simulink model "tut6_blackbox"  (Simulink 7.4)
settings: Solver=ode45  StartTime=0.0  StopTime=10.0  RelTol=1e-3
undefined symbols (not defined in the file or in its folder): gcbh, xlBlockLoadCallback
libraries: xbsIndex_r4 x4, xps_library x4, casper_library_misc x2
settings Model: Creator=jack  LastModifiedBy=jack

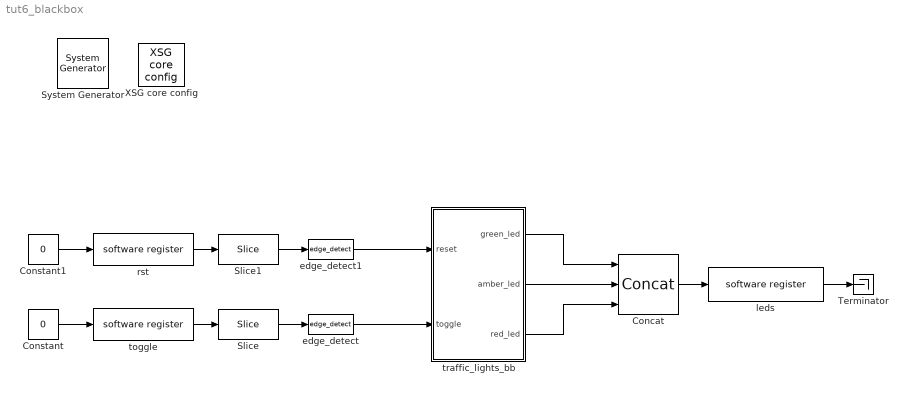
== system tut6_blackbox ==
  " System Generator" : xbsIndex_r4/ System Generator  Tag=genX  SystemSampleTime=-1  xilinxfamily=virtex5  part=xc5vsx95t  speed=-1  package=ff1136  synthesis_tool=XST  clock_wrapper=Clock Enables  directory=./tut6_blackbox/sysgen  testbench=off  simulink_period=1  sysclk_period=10  dcm_input_clock_period=100  incr_netlist=off  trim_vbits=Everywhere in SubSystem  dbl_ovrd=According to Block Masks  core_generation=According to Block Masks  run_coregen=off  deprecated_control=off  eval_field=0  block_type=sysgen
      settings: block_version=11.4
  Concat : xbsIndex_r4/Concat  num_inputs=3  dbl_ovrd=off  block_type=concat
  Constant : Constant  Value=0  OutDataType=fixdt(1, 16)  OutScaling=2^0
  Constant1 : Constant  Value=0  OutDataType=fixdt(1, 16)  OutScaling=2^0
  Slice : xbsIndex_r4/Slice  nbits=1  boolean_output=on  mode=Lower Bit Location + Width  bit1=0  base1=MSB of Input  bit0=0  base0=LSB of Input  dbl_ovrd=off  block_type=slice
  Slice1 : xbsIndex_r4/Slice  nbits=1  boolean_output=on  mode=Lower Bit Location + Width  bit1=0  base1=MSB of Input  bit0=0  base0=LSB of Input  dbl_ovrd=off  block_type=slice
  Terminator : Terminator
  XSG core config : xps_library/XSG core config  Tag=xps:xsg  SystemSampleTime=-1  hw_sys=ROACH:sx95t  ibob_linux=off  clk_src=sys_clk  iBOB_clk_src=sys_clk  BEE2_ctrl_clk_src=sys_clk  BEE2_usr_clk_src=sys_clk  ROACH_clk_src=sys_clk  ROACH2_clk_src=adc0_clk  CORR_clk_src=sys_clk  gpio_clk_io_group=iBOB:sma  gpio_clk_bit_index=0  clk_rate=100  sample_period=1  synthesis_tool=XST  mpc_type=powerpc440_ext
  edge_detect : casper_library_misc/edge_detect  SystemSampleTime=-1  edge=Rising  polarity=Active High  x_in=[0 0.08 0.08 0.16 0.16 0.24 0.24 0.32 0.32 0.4]  y_in="[-1 -1  1  1  1  1  1  1  1  1]"  x_out=[0.6 0.68 0.68 0.76 0.76 0.84 0.84 0.92 0.92 1]  y_out="[-1 -1  1  1 -1 -1 -1 -1 -1 -1]"
  edge_detect1 : casper_library_misc/edge_detect  SystemSampleTime=-1  edge=Rising  polarity=Active High  x_in=[0 0.08 0.08 0.16 0.16 0.24 0.24 0.32 0.32 0.4]  y_in="[-1 -1  1  1  1  1  1  1  1  1]"  x_out=[0.6 0.68 0.68 0.76 0.76 0.84 0.84 0.92 0.92 1]  y_out="[-1 -1  1  1 -1 -1 -1 -1 -1 -1]"
  leds : xps_library/software register  Tag=xps:sw_reg  SystemSampleTime=-1  io_dir=To Processor  arith_type=Unsigned  bitwidth=32  bin_pt=0  sample_period=1  gw_name=tut6_blackbox_leds_user_data_in
  rst : xps_library/software register  Tag=xps:sw_reg  SystemSampleTime=-1  io_dir=From Processor  arith_type=Unsigned  bitwidth=32  bin_pt=0  sample_period=1  gw_name=tut6_blackbox_rst_user_data_out
  toggle : xps_library/software register  Tag=xps:sw_reg  SystemSampleTime=-1  io_dir=From Processor  arith_type=Unsigned  bitwidth=32  bin_pt=0  sample_period=1  gw_name=tut6_blackbox_toggle_user_data_out
  traffic_lights_bb : Subsystem  mask{amber_time=200000000}
      mask prompts: amber_time "Number of amber light clock cycles?"
  wires:
  toggle/1 -> Slice/1
  Slice/1 -> edge_detect/1
  edge_detect/1 -> traffic_lights_bb/2(toggle)
  rst/1 -> Slice1/1
  Slice1/1 -> edge_detect1/1
  edge_detect1/1 -> traffic_lights_bb/1(reset)
  Concat/1 -> leds/1
  traffic_lights_bb/1(green_led) -> Concat/1
  traffic_lights_bb/2(amber_led) -> Concat/2
  traffic_lights_bb/3(red_led) -> Concat/3
  leds/1 -> Terminator/1
  Constant/1 -> toggle/1
  Constant1/1 -> rst/1

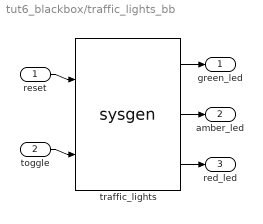
== system tut6_blackbox/traffic_lights_bb ==
  reset : Inport
  toggle : Inport  Port=2
  traffic_lights : S-Function  AncestorBlock=xbsIndex_r4/Black Box  LoadFcn=xlBlockLoadCallback(gcbh);  FunctionName=sysgen  Parameters=ptable_  EnableBusSupport=off  mask(Xilinx Black Box Block){infoedit=Incorporates black box HDL and simulation model into a System Generator design.<br><br>You must supply a Black Box with certain information about the HDL component you would like to bring into System Generator. This information is provided through a Matlab function.<br><br>When "Simulation mode" is set to "Inactive", you will typically want to provide a separate simulation model by using a Simulation Multiplexer.<br>When "Simulation mode" is set to "External co-simulator", you must include a ModelSim block in the design., init_code=traffic_lights_config, sim_method_sgadvanced=, sim_method=ISE Simulator, engine_block=, verbose=off, xl_use_area_sgadvanced=, xl_use_area=off, xl_area=[0,0,0,0,0,0,0], has_advanced_control=0, sggui_pos=1300,29,399,477, block_type=blackbox2, block_version=11.4, sg_icon_stat=105,152,2,3,white,blue,0,ffa1fd99,right,, sg_mask_display=|, sg_list_contents={'table'=>{'sim_method'=>'popup(Inactive|ISE Simulator|External co-simulator)','userSelections'=>{'sim_method'=>'ISE Simulator'}}}, sg_blockgui_xml=, amber_time=amber_time}
      mask sg_mask_display=|
      | fprintf('','COMMENT: begin icon graphics');
      | patch([0 1 1 0 ],[0 0 1 1 ],[0.77 0.82 0.91]);
      | patch([0.228571 0.0666667 0.304762 0.0666667 0.228571 0.495238 0.571429 0.647619 0.933333 0.714286 0.504762 0.352381 0.590476 0.352381 0.504762 0.714286 0.933333 0.647619 0.571429 0.495238 0.228571 ],[0.230263 0.342105 0.506579 0.671053 0.782895 0.782895 0.730263 0.782895 0.782895 0.631579 0.776316 0.671053 0.506579 0.342105 0.236842 0.381579 0.230263 0.230263 0.282895 0.230263 0.230263 ],[0.98 0.96 0.92]);
      | plot([0 1 1 0 0 ],[0 0 1 1 0 ]);
      | fprintf('','COMMENT: end icon graphics');
      | fprintf('','COMMENT: begin icon text');
      | color('black');port_label('input',1,'reset');
      | color('black');port_label('input',2,'toggle');
      | color('black');port_label('output',1,'green_led');
      | color('black');port_label('output',2,'amber_led');
      | color('black');port_label('output',3,'red_led');
      | fprintf('','COMMENT: end icon text');
      mask prompts: infoedit ""; init_code "Block configuration m-function"; sim_method_sgadvanced ""; sim_method "Simulation mode"; engine_block "HDL co-simulator to use  (specify helper block by name)"; xl_use_area_sgadvanced ""; xl_use_area "Define FPGA area for resource estimation"; xl_area "FPGA area [slices, FFs, BRAMs, LUTs, IOBs, emb. mults, TBUFs]"; has_advanced_control ""; sggui_pos ""; block_type ""; block_version ""; sg_icon_stat ""; sg_mask_display ""; sg_list_contents ""; sg_blockgui_xml ""; amber_time "Amber clock light cycles?"
      mask help:
      | Incorporates black box HDL and simulation model into a System Generator design.
      |
      | You must supply a Black Box with certain information about the HDL component you would like to bring into System Generator. This information is provided through a Matlab function.
      |
      | When "Simulation mode" is set to "Inactive", you will typically want to provide a separate simulation model by using a Simulation Multiplexer.
      | When "Simulation mode" is set to "External co-simulator", you must include a ModelSim block in the design.
      mask init:
      | try
      |   tmp_gcb = gcb;
      |   tmp_gcbh = gcbh;
      |   if (strcmp('SysGenIndex',get_param(bdroot(tmp_gcbh),'tag')) && ~isempty(regexp(bdroot(tmp_gcb), '^xbs', 'once')))
      |     return;
      |   end;
      |   xlMungeMaskParams;
      |   block_config = 'sysgen_blockset:black_box_config';
      | 
      |   block_type='blackbox2';
      | 
      |   serialized_declarations = '{''engineWorkDir''=>''String'',''engine_block''=>''String'',''engine_handle''=>''Double'',''init_code''=>''String'',''mdlPath''=>''String'',''sim_method''=>''Int'',''srcPath''=>''String'',''validEngineBlock''=>''Int'',''verbose''=>''Bool'',''block_type''=>''String''}';
      |   xlblackbox2_init();
      |   ptable_ = xlblockprep(get_param(tmp_gcb, 'MaskWSVariables'));
      | catch
      |   global dbgsysgen;
      |   if(~isempty(dbgsysgen) && dbgsysgen)
      |     e = regexprep(lasterr, '\n', '\nError: ');
      |     disp(['Error: While running MaskInit code on block ' tmp_gcb ': ' e]);
      |     error(e);
      |   end
      | end
      settings: CopyFcn=xlBlockMoveCallback(gcbh);;xlbbCopyCallback;  DeleteFcn=xlDestroyGui(gcbh);  ModelCloseFcn=xlDestroyGui(gcbh);  PreSaveFcn=xlBlockPreSaveCallback(gcbh);  PostSaveFcn=xlBlockPostSaveCallback(gcbh);  DestroyFcn=xlDestroyGui(gcbh);  OpenFcn=xlOpenGui(gcbh, 'blackbox2_gui.xml', @blackbox2enablement, -1)  CloseFcn=xlDestroyGui(gcbh);  MoveFcn=xlBlockMoveCallback(gcbh);
      mask Help: eval('');xlDoc('-book','sysgen','-topic','Black_Box');
      mask StyleString: edit,edit,edit,popup(Inactive|ISE Simulator|External co-simulator),edit,checkbox,edit,checkbox,edit,edit,edit,edit,edit,edit,edit,edit,edit,edit
      mask Display:
      | fprintf('','COMMENT: begin icon graphics');
      | patch([0 1 1 0 ],[0 0 1 1 ],[0.77 0.82 0.91]);
      | patch([0.228571 0.0666667 0.304762 0.0666667 0.228571 0.495238 0.571429 0.647619 0.933333 0.714286 0.504762 0.352381 0.590476 0.352381 0.504762 0.714286 0.933333 0.647619 0.571429 0.495238 0.228571 ],[0.230263 0.342105 0.506579 0.671053 0.782895 0.782895 0.730263 0.782895 0.782895 0.631579 0.776316 0.671053 0.506579 0.342105 0.236842 0.381579 0.230263 0.230263 0.282895 0.230263 0.230263 ],[0.98 0.96 0.92]);
      | plot([0 1 1 0 0 ],[0 0 1 1 0 ]);
      | fprintf('','COMMENT: end icon graphics');
      | fprintf('','COMMENT: begin icon text');
      | color('black');port_label('input',1,'reset');
      | color('black');port_label('input',2,'toggle');
      | color('black');port_label('output',1,'green_led');
      | color('black');port_label('output',2,'amber_led');
      | color('black');port_label('output',3,'red_led');
      | fprintf('','COMMENT: end icon text');
  green_led : Outport
  amber_led : Outport  Port=2
  red_led : Outport  Port=3
  wires:
  traffic_lights/1 -> green_led/1
  reset/1 -> traffic_lights/1
  traffic_lights/2 -> amber_led/1
  toggle/1 -> traffic_lights/2
  traffic_lights/3 -> red_led/1
